simulink subsystem "load_model"  (R2024b)
settings: Solver=VariableStepAuto  StartTime=0.0  StopTime=10.0  RelTol=1e-3
undefined symbols (not defined in the file or in its folder): Newton, Raphson
libraries: fl_lib x8, nesl_utility x4
settings Model: Creator=eric  LastModifiedBy=eric

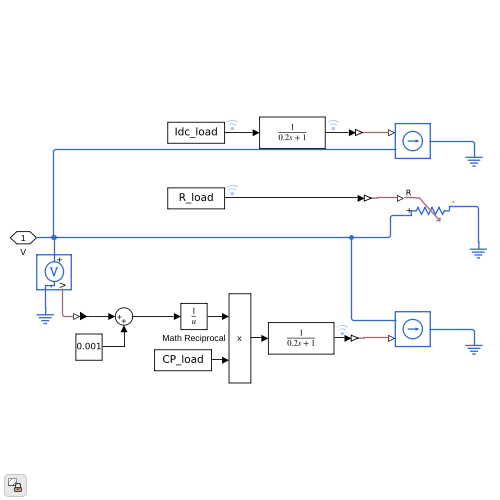
[thumbnail: Simulink's stored preview of the top-level diagram]
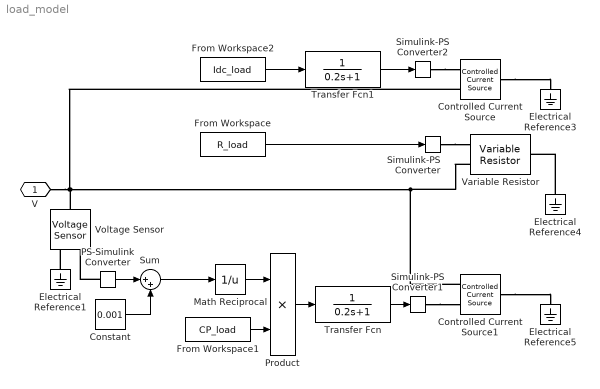
== system load_model ==
  Constant : Constant  Value=0.001
  Controlled Current Source : fl_lib/Electrical/Electrical Sources/Controlled Current Source
  Controlled Current Source1 : fl_lib/Electrical/Electrical Sources/Controlled Current Source
  Electrical Reference{1,3..5} (4 alike) : fl_lib/Electrical/Electrical Elements/Electrical Reference
  From Workspace : FromWorkspace  VariableName=R_load  OutputAfterFinalValue=Holding final value
  From Workspace1 : FromWorkspace  VariableName=CP_load  OutputAfterFinalValue=Holding final value
  From Workspace2 : FromWorkspace  VariableName=Idc_load  OutputAfterFinalValue=Holding final value
  Math Reciprocal : Math  Operator=reciprocal  AlgorithmMethod=Newton-Raphson  SignedPower=on  OutMax=0.1
  PS-Simulink Converter : nesl_utility/PS-Simulink Converter  PhysicalDomain=network_engine_domain  SubClassName=ps_output  LeftPortType=input  RightPortType=output  PseudoPeriodic=off  Frequencies=[]  VectorFormat=inherit  Unit=inherit  AffineConversion=off
  Product : Product
  Simulink-PS Converter : nesl_utility/Simulink-PS Converter  PhysicalDomain=network_engine_domain  SubClassName=ps_input  LeftPortType=input  RightPortType=output  PseudoPeriodic=off  Frequencies=[]  NoiseDistribution=none  NoiseParameters=[]  Unit=1  AffineConversion=off  FilteringAndDerivatives=provide  SimscapeFilterOrder=1  InputFilterTimeConstant=0.001  UdotUserProvided=0
  Simulink-PS Converter1 : nesl_utility/Simulink-PS Converter  PhysicalDomain=network_engine_domain  SubClassName=ps_input  LeftPortType=input  RightPortType=output  PseudoPeriodic=off  Frequencies=[]  NoiseDistribution=none  NoiseParameters=[]  Unit=1  AffineConversion=off  FilteringAndDerivatives=provide  SimscapeFilterOrder=1  InputFilterTimeConstant=0.001  UdotUserProvided=0
  Simulink-PS Converter2 : nesl_utility/Simulink-PS Converter  PhysicalDomain=network_engine_domain  SubClassName=ps_input  LeftPortType=input  RightPortType=output  PseudoPeriodic=off  Frequencies=[]  NoiseDistribution=none  NoiseParameters=[]  Unit=1  AffineConversion=off  FilteringAndDerivatives=provide  SimscapeFilterOrder=1  InputFilterTimeConstant=0.001  UdotUserProvided=0
  Sum : Sum  Inputs=|++
  Transfer Fcn : TransferFcn  Denominator=[0.2 1]
  Transfer Fcn1 : TransferFcn  Denominator=[0.2 1]
  Variable Resistor : fl_lib/Electrical/Electrical Elements/Variable Resistor  Rmin=0 Ohm  thermalEnable=false  thermal_mass=1 J/K  i_specify=off  i_priority=None  i=0 A  i_nominal_specify=off  i_nominal_value=1  i_nominal_unit=A  v_specify=off  v_priority=None  v=0 V  v_nominal_specify=off  v_nominal_value=1  v_nominal_unit=V  T_specify=off  T_priority=None  T=300 K  T_nominal_specify=off  T_nominal_value=1  T_nominal_unit=K
  Voltage Sensor : fl_lib/Electrical/Electrical Sensors/Voltage Sensor
  V : PMIOPort  Side=Left
  wires:
  Product/1 -> Transfer Fcn/1
  From Workspace1/1 -> Product/2
  Math Reciprocal/1 -> Product/1
  Transfer Fcn/1 -> Simulink-PS Converter1/1
  From Workspace/1 -> Simulink-PS Converter/1
  Constant/1 -> Sum/2
  PS-Simulink Converter/1 -> Sum/1
  Sum/1 -> Math Reciprocal/1
  From Workspace2/1 -> Transfer Fcn1/1
  Transfer Fcn1/1 -> Simulink-PS Converter2/1
  connections:
  Controlled Current Source/RConn2 -- Controlled Current Source1/RConn2 -- Variable Resistor/LConn2 -- Voltage Sensor/LConn1 -- V/RConn1
  Simulink-PS Converter/RConn1 -- Variable Resistor/LConn1
  Controlled Current Source/LConn1 -- Electrical Reference3/LConn1
  Simulink-PS Converter2/RConn1 -- Controlled Current Source/RConn1
  Electrical Reference4/LConn1 -- Variable Resistor/RConn1
  Electrical Reference1/LConn1 -- Voltage Sensor/RConn2
  PS-Simulink Converter/LConn1 -- Voltage Sensor/RConn1
  Controlled Current Source1/LConn1 -- Electrical Reference5/LConn1
  Simulink-PS Converter1/RConn1 -- Controlled Current Source1/RConn1
